simulink subsystem "OL_PTI_eSPAARO_5"  (R2025a)
settings: Solver=VariableStepAuto  StartTime=0.0  StopTime=10.0  RelTol=1e-3
undefined symbols (not defined in the file): FC
libraries: simulink x2
settings Model: Creator=gurt1  LastModifiedBy=gurt1
settings RTWCC: GPUComputeCapability=3.5

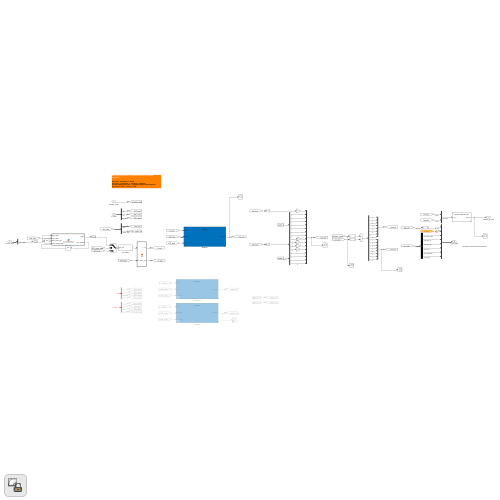
[thumbnail: Simulink's stored preview of the top-level diagram]
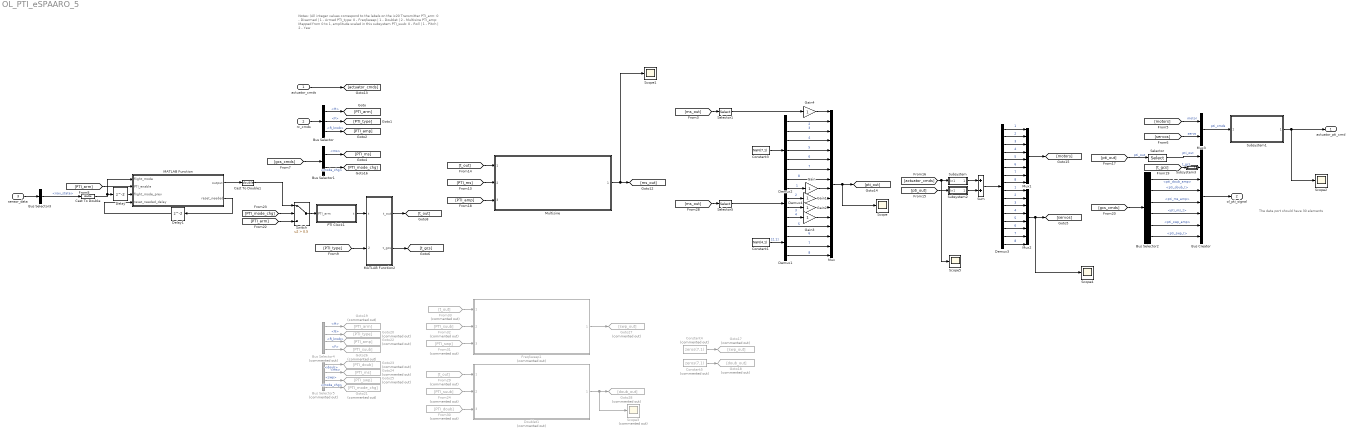
== system OL_PTI_eSPAARO_5 ==
  note: The data port should have 30 elements
  note: Notes: (All integer values correspond to the labels on the ix20 Transmitter
      |
      | PTI_arm: 0 - Disarmed | 1 - Armed
      | PTI_type: 0 - FreqSweep | 1 - Doublet | 2 - Multisine
      | PTI_amp: Mapped from 0 to 1, amplitude scaled in this subsystem
      | PTI_suub: 0 - Roll | 1 - Pitch | 2 - Yaw
  actuator_cmds : Inport
  rc_cmds : Inport  Port=2
  sensor_data : Inport  Port=3
  Bus Creator : BusCreator  Inputs=8
  Bus Selector : BusSelector  OutputSignals=switches.H,switches.F,switches.R_knob
  Bus Selector1 : BusSelector  OutputSignals=PTI.PTI.ms,PTI.PTI.mode_chg
  Bus Selector2 : BusSelector  OutputSignals=PTI.PTI.doub.pti_doub_amp,PTI.PTI.doub.pti_doub_t,PTI.PTI.ms.pti_ms_amp,PTI.PTI.ms.pti_ms_t,PTI.PTI.swp.pti_swp_amp,PTI.PTI.swp.pti_swp_t
  Bus Selector3 : BusSelector  OutputSignals=nav_state
  Bus Selector4 : BusSelector  Commented=on  OutputSignals=switches.H,switches.G,switches.R_knob,switches.F
  Bus Selector5 : BusSelector  Commented=on  OutputSignals=PTI.PTI.doub,PTI.PTI.ms,PTI.PTI.swp,PTI.PTI.mode_chg
  Cast To Double : DataTypeConversion  OutDataTypeStr=double  SaturateOnIntegerOverflow=off  RndMeth=Floor
  Cast To Double1 : DataTypeConversion  OutDataTypeStr=double  SaturateOnIntegerOverflow=off  RndMeth=Floor
  Constant1 : Constant  Value=NaN(4,1)
  Constant3 : Constant  Value=NaN(7,1)
  Constant4 : Constant  Commented=on  Value=zeros(7,1)  SampleTime=-1
  Constant5 : Constant  Commented=on  Value=zeros(7,1)  SampleTime=-1
  Delay : Delay
  Delay1 : Delay
  Demux1 : Demux
  Demux2 : Demux  Outputs=7
  Demux3 : Demux  Outputs=16
  Demux4 : Demux
  Doublet1 : Subsystem  Commented=on  ReferencedSubsystem=Doublet
  FreqSweep1 : Subsystem  Commented=on  ReferencedSubsystem=FreqSweep
  From24 : From  Commented=on  GotoTag=PTI_suub
  From29 : From  Commented=on  GotoTag=t_out
  From30 : From  Commented=on  GotoTag=PTI_doub
  From31 : From  Commented=on  GotoTag=PTI_swp
  From32 : From  Commented=on  GotoTag=PTI_suub
  From33 : From  Commented=on  GotoTag=t_out
  Gain{,1..4} (5 alike) : Gain
  Goto17 : Goto  Commented=on  GotoTag=swp_out
  Goto18 : Goto  Commented=on  GotoTag=doub_out
  Goto19 : Goto  Commented=on  GotoTag=PTI_arm
  Goto20 : Goto  Commented=on  GotoTag=PTI_type
  Goto21 : Goto  Commented=on  GotoTag=PTI_mode_chg
  Goto22 : Goto  Commented=on  GotoTag=PTI_amp
  Goto23 : Goto  Commented=on  GotoTag=PTI_doub
  Goto24 : Goto  Commented=on  GotoTag=PTI_ms
  Goto25 : Goto  Commented=on  GotoTag=PTI_swp
  Goto26 : Goto  Commented=on  GotoTag=PTI_suub
  Goto27 : Goto  Commented=on  GotoTag=swp_out
  Goto28 : Goto  Commented=on  GotoTag=doub_out
  MATLAB Function : MATLAB Function  TreatAsAtomicUnit=on
  MATLAB Function2 : MATLAB Function  TreatAsAtomicUnit=on
  Multisine : Subsystem  ReferencedSubsystem=Multisine
  Mux : Mux  Inputs=16
  Mux1 : Mux  Inputs=8
  Mux2 : Mux  Inputs=8
  Mux3 : Mux  Inputs=2
  PTI Clock1 : Subsystem
  Scope{,1..2,4..5} (5 alike) : Scope
      Scope settings: ActiveDisplayYMinimum=-1.3876149166777767  ActiveDisplayYMaximum=0.55989998750313119  DataLoggingVariableName=ScopeData9
      Scope1 settings: ActiveDisplayYMinimum=-1.201025703337677  ActiveDisplayYMaximum=1.1721816821342206  DataLoggingVariableName=ScopeData14
      Scope2 settings: ActiveDisplayYMinimum=-0.38806971868771378  ActiveDisplayYMaximum=0.78783850310960957  DataLoggingVariableName=ScopeData15
      Scope4 settings: ActiveDisplayYMinimum=-0.48752197265624941  ActiveDisplayYMaximum=1.3209252929687505  DataLoggingVariableName=ScopeData17
      Scope5 settings: ActiveDisplayYMinimum=-3.5416479492187491  ActiveDisplayYMaximum=2.9333520507812505  DataLoggingVariableName=ScopeData18
  Scope3 : Scope  Commented=on
      settings: ActiveDisplayYMinimum=-1  ActiveDisplayYMaximum=1  DataLoggingVariableName=ScopeData16
  Selector : Selector  InputPortWidth=16  IndexOptions=Index vector (dialog)  Indices=[1,9:14]  OutputSizes=1
  Selector1 : Selector  InputPortWidth=5  IndexOptions=Index vector (dialog)  Indices=1  OutputSizes=1
  Selector5 : Selector  InputPortWidth=5  IndexOptions=Index vector (dialog)  Indices=[2:5]  OutputSizes=1
  Subsystem : Subsystem
  Subsystem1 : Subsystem  ReferencedSubsystem=Actuator_Manual_Cmd
  Subsystem2 : Subsystem
  Subsystem3 : Subsystem
  Sum : Sum
  Switch : Switch  Criteria=u2 > Threshold  Threshold=0.5  SaturateOnIntegerOverflow=off  InputSameDT=off
  actuator_pti_cmd : Outport
  ol_pti_signal : Outport  Port=2
  wires:
  Selector/1 -> Bus Creator/1  "pti_out"
  Constant5/1 -> Goto18/1
  Constant4/1 -> Goto17/1
  Demux4/4 -> Gain3/1  "4"
  Demux2/7 -> Mux/8  "8"
  Demux2/6 -> Mux/7  "7"
  Demux2/5 -> Mux/6  "6"
  Demux2/4 -> Mux/5  "5"
  Demux2/3 -> Mux/4  "4"
  Demux2/2 -> Mux/3  "3"
  Demux2/1 -> Mux/2  "2"
  Selector5/1 -> Demux4/1
  [PTI_type] -> MATLAB Function2/2(PTI_type)
  Subsystem3/1(Out1) -> Bus Creator/2
  [t_gcs] -> Subsystem3/1(In1)  "t_gcs"
  Demux3/7 -> Mux1/7  "7"
  Subsystem2/1(Out1) -> Sum/2
  Subsystem/1(Out1) -> Sum/1
  [ms_out] -> Selector5/1
  Demux4/2 -> Gain1/1  "2"
  Demux4/1 -> Gain/1  "1"
  Demux4/3 -> Gain2/1  "3"
  Constant3/1 -> Demux2/1
  Bus Selector3/1 -> Cast To Double/1  "<nav_state>"
  sensor_data/1 -> Bus Selector3/1
  MATLAB Function/1(output) -> Cast To Double1/1
  Delay1/1 -> MATLAB Function/4(reset_needed_delay)
  MATLAB Function/2(reset_needed) -> Delay1/1
  [PTI_arm] -> MATLAB Function/2(PTI_enable)
  Delay/1 -> MATLAB Function/3(flight_mode_prev)
  Cast To Double/1 -> Delay/1, MATLAB Function/1(flight_mode)
  Bus Selector/1 -> [PTI_arm]  "<H>"
  Demux3/12 -> Mux2/4  "4"
  [gcs_cmds] -> Bus Selector1/1
  Mux3/1 -> Subsystem1/1  "pti_cmds"
  [servos] -> Mux3/2  "servo"
  [motors] -> Mux3/1  "motor"
  Bus Creator/1 -> ol_pti_signal/1
  rc_cmds/1 -> Bus Selector/1
  Bus Selector/3 -> [PTI_amp]  "<R_knob>"
  Bus Selector1/1 -> [PTI_ms]  "<ms>"
  Cast To Double1/1 -> Switch/1
  PTI Clock1/1(t) -> MATLAB Function2/1(t)
  MATLAB Function2/1(t_out) -> [t_out]
  [t_out] -> Multisine/1
  [PTI_ms] -> Multisine/2
  Multisine/1 -> [ms_out], Scope1/1
  [ms_out] -> Selector1/1
  actuator_cmds/1 -> [actuator_cmds]
  Mux/1 -> [pti_out], Scope/1
  [pti_out] -> Subsystem2/1(In1)
  [actuator_cmds] -> Scope5/1, Subsystem/1(In1)
  Sum/1 -> Demux3/1
  Demux3/1 -> Mux1/1  "1"
  Demux3/2 -> Mux1/2  "2"
  Demux3/3 -> Mux1/3  "3"
  Demux3/4 -> Mux1/4  "4"
  Demux3/5 -> Mux1/5  "5"
  Demux3/6 -> Mux1/6  "6"
  Demux3/8 -> Mux1/8  "8"
  Demux3/14 -> Mux2/6  "6"
  Demux3/15 -> Mux2/7  "7"
  Demux3/13 -> Mux2/5  "5"
  Demux3/16 -> Mux2/8  "8"
  Demux3/9 -> Mux2/1  "1"
  Demux3/10 -> Mux2/2  "2"
  Demux3/11 -> Mux2/3  "3"
  Mux1/1 -> [motors]
  Mux2/1 -> Scope4/1, [servos]
  [pti_out] -> Selector/1  "pti_out"
  MATLAB Function2/2(t_gcs) -> [t_gcs]
  [gcs_cmds] -> Bus Selector2/1
  Bus Selector2/1 -> Bus Creator/3  "<pti_doub_amp>"
  Bus Selector2/2 -> Bus Creator/4  "<pti_doub_t>"
  Bus Selector2/3 -> Bus Creator/5  "<pti_ms_amp>"
  Bus Selector2/4 -> Bus Creator/6  "<pti_ms_t>"
  Bus Selector2/5 -> Bus Creator/7  "<pti_swp_amp>"
  Bus Selector2/6 -> Bus Creator/8  "<pti_swp_t>"
  Subsystem1/1 -> Scope2/1, actuator_pti_cmd/1
  [PTI_arm] -> Switch/3
  Switch/1 -> PTI Clock1/1(PTI_arm)
  Bus Selector1/2 -> [PTI_mode_chg]  "<mode_chg>"
  [PTI_mode_chg] -> Switch/2
  Constant1/1 -> Demux1/1  "[2,1]"
  Bus Selector5/4 -> Goto21/1  "<mode_chg>"
  Bus Selector4/4 -> Goto26/1  "<F>"
  Bus Selector5/2 -> Goto24/1  "<ms>"
  Bus Selector5/1 -> Goto23/1  "<doub>"
  Bus Selector5/3 -> Goto25/1  "<swp>"
  Bus Selector4/3 -> Goto22/1  "<R_knob>"
  Bus Selector4/2 -> Goto20/1  "<G>"
  ? -> Bus Selector4/1
  ? -> Bus Selector5/1
  Bus Selector4/1 -> Goto19/1  "<H>"
  From32/1 -> FreqSweep1/2
  Doublet1/1 -> Scope3/1, Goto28/1
  From24/1 -> Doublet1/2
  From29/1 -> Doublet1/1
  From30/1 -> Doublet1/3
  From33/1 -> FreqSweep1/1
  From31/1 -> FreqSweep1/3
  FreqSweep1/1 -> Goto27/1
  Selector1/1 -> Gain4/1
  [PTI_amp] -> Multisine/3
  Bus Selector/2 -> [PTI_type]  "<F>"
  Demux1/1 -> Mux/13  "5"
  Demux1/2 -> Mux/14  "6"
  Demux1/3 -> Mux/15  "7"
  Demux1/4 -> Mux/16  "8"
  Gain/1 -> Mux/9
  Gain1/1 -> Mux/10
  Gain2/1 -> Mux/11
  Gain3/1 -> Mux/12
  Gain4/1 -> Mux/1

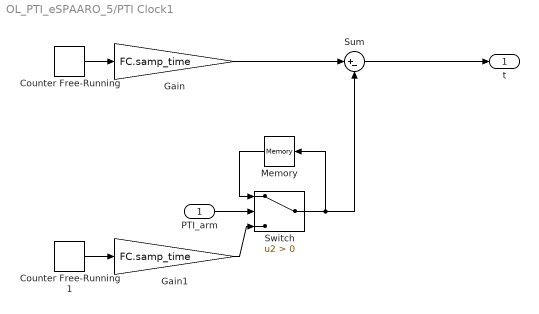
== system OL_PTI_eSPAARO_5/PTI Clock1 ==
  PTI_arm : Inport
  Counter Free-Running : simulink/Sources/Counter Free-Running  NumBits=32  tsamp=-1
  Counter Free-Running1 : simulink/Sources/Counter Free-Running  NumBits=32  tsamp=-1
  Gain : Gain  Gain=FC.samp_time  OutDataTypeStr=double
  Gain1 : Gain  Gain=FC.samp_time  OutDataTypeStr=double
  Memory : Memory
  Sum : Sum  Inputs=|+-
  Switch : Switch  Criteria=u2 > Threshold  SaturateOnIntegerOverflow=off  InputSameDT=off
  t : Outport
  wires:
  Sum/1 -> t/1
  PTI_arm/1 -> Switch/2
  Memory/1 -> Switch/1
  Switch/1 -> Memory/1, Sum/2
  Gain1/1 -> Switch/3
  Counter Free-Running1/1 -> Gain1/1
  Gain/1 -> Sum/1
  Counter Free-Running/1 -> Gain/1

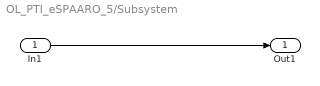
== system OL_PTI_eSPAARO_5/Subsystem ==
  In1 : Inport  PortDimensions=[16,1]
  Out1 : Outport  PortDimensions=[16,1]
  wires:
  In1/1 -> Out1/1

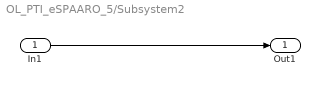
== system OL_PTI_eSPAARO_5/Subsystem2 ==
  In1 : Inport  PortDimensions=[16,1]
  Out1 : Outport  PortDimensions=[16,1]
  wires:
  In1/1 -> Out1/1

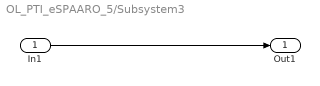
== system OL_PTI_eSPAARO_5/Subsystem3 ==
  In1 : Inport  PortDimensions=[1 1]
  Out1 : Outport  PortDimensions=[1 1]
  wires:
  In1/1 -> Out1/1

== matlab function OL_PTI_eSPAARO_5/MATLAB Function ==
  data: flight_mode input; output output; PTI_enable input; flight_mode_prev input; reset_needed_delay input; reset_needed output
function [output,reset_needed] = checkFlightMode(flight_mode, PTI_enable, flight_mode_prev, reset_needed_delay)
    % Output true (1) if flight_mode has not changed since PTI_enable was enabled
    
    % Initialize output
    output = 0;
    reset_needed = 0;

    % Take care of reset_needed if applicable
    if reset_needed_delay == 1
        if PTI_enable == 1
            reset_needed = 1;
            output = 0;
            return
        end
    end
    
    % Check if PTI_enable is off
    if PTI_enable == 1
        output = 1;
    end

    % Check if PTI_enable is on and flight_mode has changed
    if flight_mode ~= flight_mode_prev && reset_needed == 0
        output = 0;
        reset_needed = 1;
    end
end

== matlab function OL_PTI_eSPAARO_5/MATLAB Function2 ==
  data: t input; t_out output; PTI_type input; t_gcs output
function [t_out,t_gcs] = fcn(t, PTI_type)

t_gcs = t;

if PTI_type == 0
    t_out = [t,0,0];
elseif PTI_type == 1
    t_out = [0,t,0];
elseif PTI_type == 2
    t_out = [0,0,t];
else
    t_out = [0,0,0];
end
